simulink model "RedCrane_kinematic_model"  (R2024a)
settings: Solver=FixedStepAuto  StartTime=0.0  StopTime=20  FixedStep=Ts  MaxStep=0.005  RelTol=1e-3
values from neighbouring files (symbols this model uses):
  M = [1, 0, 0, (L5 + L4 - L1) ... (first row only)    [enviroment_setup.m]
  SList = [ws_mat ... (first row only)    [enviroment_setup.m]
  telescope0 = 0    [enviroment_setup.m]
  thetaList0 = [0, 0,-pi/8, 0, 0]'    [enviroment_setup.m]
  Ts = 0.001    [enviroment_setup.m]
undefined symbols (not defined in the file or in its folder): dp_k_angle_to_stroke, dp_m_angle_to_stroke, p_k_angle_to_stroke, p_k_stroke_to_angle, p_m_angle_to_stroke, p_m_stroke_to_angle, X, Y, Z
libraries: sm_lib x82, nesl_utility x19, fl_lib x16
(part 1 of 3)
settings Model: Creator=sindr  LastModifiedBy=larso
settings RTWCC: GPUComputeCapability=3.5
settings ConfigComp: PLC_OutputDir=plc_export\FB_InverceKinematics  PLC_TargetIDE=twincat3  PLC_MultiTBSigbuilderTimeRange=off  PLC_FoldFBCallOutputVar=off  PLC_RemoveUnusedSSMethodCallArguments=off  PLC_UseCallOutputArgSyntax=off  PLC_EnableUnsignedAndDoubleTypes=off  PLC_EnableUDTSplitting=off  PLC_MaxFieldsInUDT=500  PLC_InlineEnumCastFunction=off

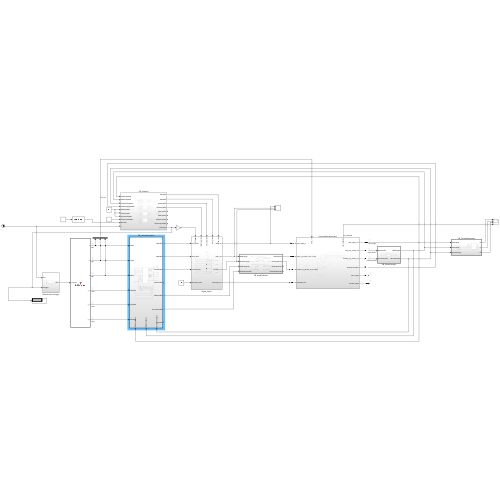
[thumbnail: Simulink's stored preview of the top-level diagram]
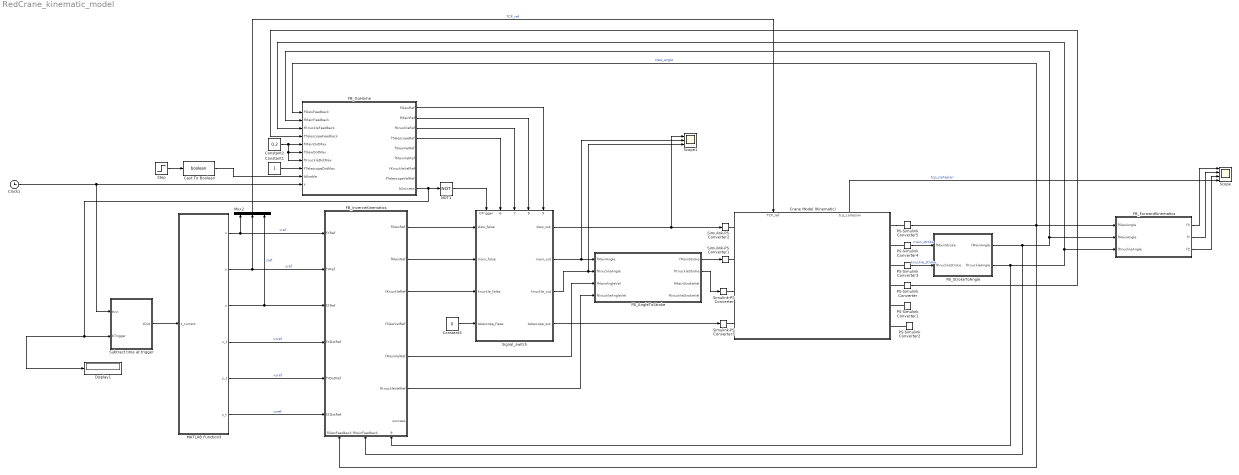
== system RedCrane_kinematic_model ==
  Cast To Boolean : DataTypeConversion  OutDataTypeStr=boolean  SaturateOnIntegerOverflow=off  RndMeth=Floor
  Clock1 : Clock
  Constant1 : Constant
  Constant2 : Constant  Value=0.2
  Constant3 : Constant  Value=0
  Crane Model (Kinematic) : Subsystem
      settings: PortSchema="{\"entries\":[{\"content\":{\"sides\":[{\"content\":{\"connectorIds\":[\"LConn1\",\"LConn2\",\"LConn3\",\"LConn4\"]},\"type\":\"ConnectorPlacement.EquallySpacedRectSide\",\"uuid\":\"4a665765-5f1a-426d-91c2-f3af20fe3627\"},{\"content\":{\"connectorIds\":[\"RConn1\",\"RConn2\",\"RConn3\",\"RConn4\",\"RConn5\",\"RConn6\"],\"side\":\"RIGHT\"},\"type\":\"ConnectorPlacement.EquallySpacedRectSide\",\"uuid\":\"cf43645c-9a50-4bc9-b355-f38e72b1430d\"},{\"content\":{\"connectorIds\":[\"In1\",\"Out1\"],\"side\":\"TOP\"},\"type\":\"ConnectorPlacement.EquallySpacedRectSide\",\"uuid\":\"253dbb23-7a12-4bfe-bf07-7d8403188f09\"}]},\"type\":\"ConnectorPlacement.EquallySpacedConnector\",\"uuid\":\"5ffb1dcc-76b9-4b5c-ba8f-4653fe2f07c9\"}],\"packageUris\":[\"http://schema.mathworks.com/mf0/Connector/R2020b\"],\"version\":\"1.0\"}"
  Display1 : Display
  FB_AngleToStroke : Subsystem  TreatAsAtomicUnit=on
  FB_ForwardKinematics : Subsystem  TreatAsAtomicUnit=on
  FB_GoHome : Subsystem
  FB_InverceKinematics : Subsystem  TreatAsAtomicUnit=on
      settings: PortSchema="{\"entries\":[{\"content\":{\"sides\":[{\"content\":{\"connectorIds\":[\"In1\",\"In2\",\"In3\",\"In4\",\"In5\",\"In6\"]},\"type\":\"ConnectorPlacement.EquallySpacedRectSide\",\"uuid\":\"b7f3f39a-cc1b-4519-b948-004466b4d293\"},{\"content\":{\"connectorIds\":[\"Out1\",\"Out2\",\"Out3\",\"Out4\",\"Out5\",\"Out6\",\"Out7\"],\"side\":\"RIGHT\"},\"type\":\"ConnectorPlacement.EquallySpacedRectSide\",\"uuid\":\"cf571c2f-2cc7-4d1d-bbc1-a75d80a0878e\"},{\"content\":{\"side\":\"TOP\"},\"type\":\"ConnectorPlacement.EquallySpacedRectSide\",\"uuid\":\"3f697bd9-7750-4474-8da5-1be48ba53c7e\"},{\"content\":{\"connectorIds\":[\"In7\",\"In8\",\"In9\"],\"side\":\"BOTTOM\"},\"type\":\"ConnectorPlacement.EquallySpacedRectSide\",\"uuid\":\"03fa0a4e-eedb-4a48-8076-446c86a2b4f7\"}]},\"type\":\"ConnectorPlacement.EquallySpacedConnector\",\"uuid\":\"6732c767-80e6-425f-b878-60bd961dd78b\"}],\"packageUris\":[\"http://schema.mathworks.com/mf0/Connector/R2020b\"],\"version\":\"1.0\"}"
  FB_StrokeToAngle : Subsystem  TreatAsAtomicUnit=on
  MATLAB Function3 : MATLAB Function  TreatAsAtomicUnit=on
  Mux2 : Mux  Inputs=3
  NOT1 : Logic  Operator=NOT  IconShape=distinctive  AllPortsSameDT=off  OutDataTypeStr=boolean
  PS-Simulink Converter{,1..5} (6 alike) : nesl_utility/PS-Simulink Converter  PhysicalDomain=network_engine_domain  SubClassName=ps_output  LeftPortType=input  RightPortType=output  PseudoPeriodic=off  Frequencies=[]  VectorFormat=inherit  Unit=inherit  AffineConversion=off
  Scope : Scope  NumInputPorts=4
  Scope1 : Scope  NumInputPorts=3
  Signal_switch : Subsystem
      settings: PortSchema="{\"entries\":[{\"content\":{\"sides\":[{\"content\":{\"connectorIds\":[\"In1\",\"In2\",\"In3\",\"In4\"]},\"type\":\"ConnectorPlacement.EquallySpacedRectSide\",\"uuid\":\"677999b9-dfe1-4592-affa-fb9b7d257ea0\"},{\"content\":{\"connectorIds\":[\"Out1\",\"Out2\",\"Out3\",\"Out4\"],\"side\":\"RIGHT\"},\"type\":\"ConnectorPlacement.EquallySpacedRectSide\",\"uuid\":\"3f36c443-9717-41bf-801d-3d95a9d66f59\"},{\"content\":{\"connectorIds\":[\"In5\",\"In6\",\"In7\",\"In8\",\"In9\"],\"side\":\"TOP\"},\"type\":\"ConnectorPlacement.EquallySpacedRectSide\",\"uuid\":\"b7ea9b48-8dcd-4abb-ae26-aa1832701a6a\"}]},\"type\":\"ConnectorPlacement.EquallySpacedConnector\",\"uuid\":\"7d55d43f-82cc-482c-a650-cc44ad6cee22\"}],\"packageUris\":[\"http://schema.mathworks.com/mf0/Connector/R2020b\"],\"version\":\"1.0\"}"
  Simulink-PS Converter{,1..3} (4 alike) : nesl_utility/Simulink-PS Converter  PhysicalDomain=network_engine_domain  SubClassName=ps_input  LeftPortType=input  RightPortType=output  PseudoPeriodic=off  Frequencies=[]  NoiseDistribution=none  NoiseParameters=[]  Unit=1  AffineConversion=off  FilteringAndDerivatives=filter  SimscapeFilterOrder=2  InputFilterTimeConstant=0.001  UdotUserProvided=0
  Step : Step  SampleTime=0
  Subtract time at trigger : Subsystem
  wires:
  FB_AngleToStroke/2(fKnuckleStroke) -> Simulink-PS Converter/1
  Mux2/1 -> Crane Model (Kinematic)/1(TCP_ref)  "TCP_ref"
  PS-Simulink Converter5/1 -> FB_InverceKinematics/7(fSlewFeedback), FB_ForwardKinematics/1(fSlewAngle), FB_GoHome/1(fSlewFeedback)  "slew_angle"
  PS-Simulink Converter/1 -> FB_GoHome/4(fTelescopeFeedback)
  Constant2/1 -> FB_GoHome/5(fMainDotMax), FB_GoHome/7(fKnuckleDotMax), FB_GoHome/6(fSlewDotMax)
  Cast To Boolean/1 -> FB_GoHome/9(bEnable)
  Step/1 -> Cast To Boolean/1
  FB_GoHome/9(bSuccess) -> NOT1/1, Display1/1, Subtract time at trigger/2(bTrigger)
  Constant1/1 -> FB_GoHome/8(fTelescopeDotMax)
  Clock1/1 -> FB_GoHome/10(t), Subtract time at trigger/1(tInn)
  Subtract time at trigger/1(tOut) -> MATLAB Function3/1(t_current)
  FB_StrokeToAngle/2(fKnuckleAngle) -> FB_GoHome/3(fKnuckleFeedback), FB_ForwardKinematics/3(fKnuckleAngle), FB_InverceKinematics/9(fKnuckleFeedback)
  FB_StrokeToAngle/1(fMainAngle) -> FB_GoHome/2(fMainFeedback), FB_ForwardKinematics/2(fMainAngle), FB_InverceKinematics/8(fMainFeedback)
  PS-Simulink Converter4/1 -> FB_StrokeToAngle/1(fMainStroke)  "main_stroke"
  PS-Simulink Converter3/1 -> FB_StrokeToAngle/2(fKnuckleStroke)  "knuckle_stroke"
  FB_InverceKinematics/5(fMainVelRef) -> FB_AngleToStroke/3(fMainAngleVel)
  FB_InverceKinematics/6(fKnuckleVelRef) -> FB_AngleToStroke/4(fKnuckleAngleVel)
  FB_GoHome/1(fSlewRef) -> Signal_switch/9(slew_true)
  FB_GoHome/2(fMainRef) -> Signal_switch/8(main_true)
  FB_GoHome/3(fKnuckleRef) -> Signal_switch/7(knuckle_true)
  FB_GoHome/4(fTelescopeRef) -> Signal_switch/6(telescope_true)
  NOT1/1 -> Signal_switch/5(bTrigger)
  FB_InverceKinematics/1(fSlewRef) -> Signal_switch/1(slew_false)
  FB_InverceKinematics/2(fMainRef) -> Signal_switch/2(main_false)
  FB_InverceKinematics/3(fKnuckleRef) -> Signal_switch/3(knuckle_false)
  Constant3/1 -> Signal_switch/4(telescope_flase)
  Signal_switch/1(slew_out) -> Scope1/1, Simulink-PS Converter2/1
  Signal_switch/2(main_out) -> Scope1/2, FB_AngleToStroke/1(fMainAngle)
  Signal_switch/3(knuckle_out) -> Scope1/3, FB_AngleToStroke/2(fKnuckleAngle)
  Signal_switch/4(telescope_out) -> Simulink-PS Converter3/1
  FB_AngleToStroke/1(fMainStroke) -> Simulink-PS Converter1/1
  MATLAB Function3/1(x) -> Mux2/1, FB_InverceKinematics/1(fXRef)  "xref"
  MATLAB Function3/2(y) -> FB_InverceKinematics/2(fYRef), Mux2/2  "yref"
  MATLAB Function3/3(z) -> Mux2/3, FB_InverceKinematics/3(fZRef)  "zref"
  MATLAB Function3/4(x_t) -> FB_InverceKinematics/4(fXDotRef)  "vxref"
  MATLAB Function3/5(y_t) -> FB_InverceKinematics/5(fYDotRef)  "vyref"
  MATLAB Function3/6(z_t) -> FB_InverceKinematics/6(fZDotRef)  "vzref"
  FB_ForwardKinematics/1(fX) -> Scope/1
  FB_ForwardKinematics/2(fY) -> Scope/2
  FB_ForwardKinematics/3(fZ) -> Scope/3
  Crane Model (Kinematic)/1(tcp_cartesian) -> Scope/4  "tcp_cartesian"
  connections:
  Simulink-PS Converter/RConn1 -- Crane Model (Kinematic)/LConn3
  Simulink-PS Converter2/RConn1 -- Crane Model (Kinematic)/LConn1
  Simulink-PS Converter1/RConn1 -- Crane Model (Kinematic)/LConn2
  Simulink-PS Converter3/RConn1 -- Crane Model (Kinematic)/LConn4
  PS-Simulink Converter/LConn1 -- Crane Model (Kinematic)/RConn4
  PS-Simulink Converter1/LConn1 -- Crane Model (Kinematic)/RConn5
  PS-Simulink Converter2/LConn1 -- Crane Model (Kinematic)/RConn6
  PS-Simulink Converter3/LConn1 -- Crane Model (Kinematic)/RConn3
  PS-Simulink Converter4/LConn1 -- Crane Model (Kinematic)/RConn2
  Crane Model (Kinematic)/RConn1 -- PS-Simulink Converter5/LConn1
